simulink model "BALLBOT_2"  (R2015a)
settings: Solver=ode45  SolverMode=SingleTasking  StartTime=0  StopTime=90  MaxStep=0.001  RelTol=1e-3  AbsTol=1e-6
InitFcn:
  | parametros;
StartFcn:
  | %vrview('Ballbot2')
StopFcn:
  | graficos;
values from neighbouring files (symbols this model uses):
  g = 9.81    [parametros.m]
  Ic = 0.024    [parametros.m]
  L = 0.2    [parametros.m]
  Mc = 1.6    [parametros.m]
  Mr = 0.5    [parametros.m]
  r = 0.12    [parametros.m]
undefined symbols (not defined in the file or in its folder): K
libraries: vrlib x4, mblibv1 x1
settings Model: ExtModeAutoUpdateStatusClock=off  Creator=The MathWorks Inc.  LastModifiedBy=Pedro
settings DataIOCC: ExternalInput=[]  InitialState=[]  LimitDataPoints=off  SignalLoggingSaveFormat=ModelDataLogs  SaveOutput=off  SaveTime=off
settings OptimizationCC: BlockReduction=off  BooleanDataType=off  BufferReuse=off  ExpressionDepthLimit=2147483647  InitFltsAndDblsToZero=on
settings DebuggingCC: AlgebraicLoopMsg=none  SaveWithParameterizedLinksMsg=none  UnderspecifiedInitializationDetection=Classic  MergeDetectMultiDrivingBlocksExec=none  SignalResolutionControl=TryResolveAllWithWarning  MultiTaskDSMMsg=warning  MultiTaskCondExecSysMsg=none  SigSpecEnsureSampleTimeMsg=none  FcnCallInpInsideContextMsg=UseLocalSettings  UnconnectedInputMsg=none  UnconnectedOutputMsg=none  UnconnectedLineMsg=none  StateNameClashWarn=warning
settings HardwareCC: TargetLongLongMode=on  TargetIntDivRoundTo=Zero  TargetEndianess=LittleEndian  TargetHWDeviceType=MATLAB Host  ProdEqTarget=off
settings GRTTargetCC: TargetFcnLib=ansi_tfl_tmw.mat  CombineOutputUpdateFcns=off  GRTInterface=on

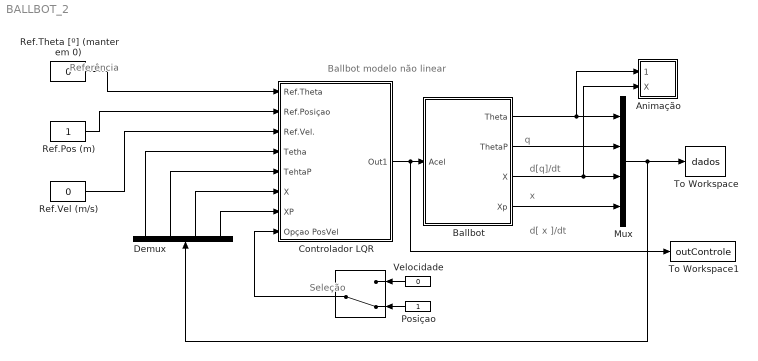
== system BALLBOT_2 ==
  note: Ballbot modelo não linear
  note: Referência
  note: Seleção
  note: x
  note: d[ x ]/dt
  note: q
  note: d[q]/dt
  " " : ManualSwitch  CurrentSetting=0
  "Animação " : Subsystem
  Ballbot : Subsystem  mask(Ballbot){thetac0=0}
      mask prompts: thetac0 "Ângulo inicial do corpo (graus)"
      mask help:
      | Modelo dinâmico não-linear do Ballbot.
      | Selecione "Look Under Mask" para ver o diagrama de simulação.
      mask Help: Unmask and double-click to see dynamics.
      mask Display: image(imread('ballbot_LMI.png'));
  Controlador LQR : Subsystem
      mask Display:
      | image(imread('ArduinoMega.png'));
      | 
      | 
      | 
      | port_label('output', 1, 'Acel Ang.');
      | 
      | port_label('input', 1, 'Ref.Theta');
      | port_label('input', 2, 'Ref.Pos.');
      | port_label('input', 3, 'Ref.Vel.');
      | port_label('input', 4, 'Theta');
      | port_label('input', 5, 'ThetaP');
      | port_label('input', 6, 'X');
      | port_label('input', 7, 'XP');
      | 
      | port_label('input', 8, 'Opção Pos.Vel');
  Demux : Demux
  Mux : Mux
  Posiçao : Constant
  "Ref.Pos (m) " : Constant
  Ref.Theta [º] (manter em 0) : Constant  Value=0
  Ref.Vel (m/s) : Constant  Value=0
  To Workspace : ToWorkspace  VariableName=dados  SaveFormat=Structure With Time  SampleTime=-1
  To Workspace1 : ToWorkspace  VariableName=outControle  SaveFormat=Structure With Time  SampleTime=-1
  Velocidade : Constant  Value=0
  wires:
  Ballbot/1(Theta) -> "Animação "/1("Pitch "), Mux/1
  Ballbot/2(ThetaP) -> Mux/2
  Ballbot/4(Xp) -> Mux/4
  Ref.Theta [º] (manter em 0)/1 -> Controlador LQR/1(Ref.Theta)
  Ref.Vel (m/s)/1 -> Controlador LQR/3(Ref.Vel.)
  Demux/1 -> Controlador LQR/4(Tetha)
  Demux/2 -> Controlador LQR/5(TehtaP)
  Demux/3 -> Controlador LQR/6(X)
  Demux/4 -> Controlador LQR/7(XP)
  Mux/1 -> Demux/1, To Workspace/1
  Velocidade/1 -> " "/1
  Posiçao/1 -> " "/2
  " "/1 -> Controlador LQR/8(Opçao PosVel)
  "Ref.Pos (m) "/1 -> Controlador LQR/2(Ref.Posiçao)
  Controlador LQR/1(Out1) -> To Workspace1/1, Ballbot/1(Acel)
  Ballbot/3(X) -> "Animação "/2(X), Mux/3

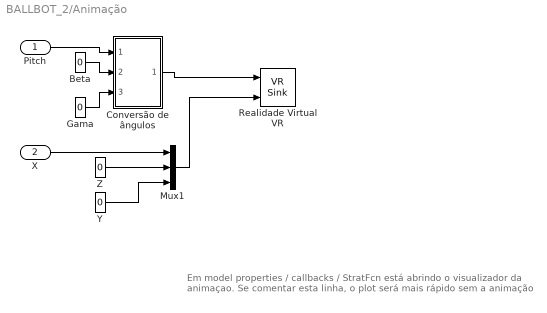
== system BALLBOT_2/Animação  ==
  note: Em model properties / callbacks / StratFcn está abrindo o visualizador da animaçao. Se comentar esta linha, o plot será mais rápido sem a animação
  "Pitch " : Inport
  X : Inport  Port=2
  Beta : Constant  Value=0
  Conversão de ângulos : Subsystem
  Gama : Constant  Value=0
  Mux1 : Mux  Inputs=3
  Realidade Virtual VR : vrlib/VR Sink  InstantiateOnLoad=on  SampleTime=0.001  ViewEnable=on  RemoteChange=off  RemoteView=off  FieldsWritten=Ballbot.rotation.4.1.1.double#Ballbot.translation.3.1.1.double  WorldFileName=Ballbot2.WRL  AutoView=on  VideoDimensions=[]  AllowVariableSize=off  FigureProperties="{'Position', 'Name', 'Viewpoint', 'CameraBound', 'CameraDirection', 'CameraPosition', 'CameraUpVector', 'ZoomFactor', 'Antialiasing', 'Headlight', 'Lighting', 'NavPanel', 'Sound', 'StatusBar', 'Stereo3D', 'Stereo3DCameraOffset', 'Stereo3DHIT', 'ToolBar', 'Textures', 'Transparency', 'Triad', 'Wireframe', 'NavZones', 'NavMode', 'NavSpeed', 'CaptureFileFormat', 'CaptureFileName', 'Record2DCompressMethod', 'Record2DCompressQuality', 'Record2D', 'Record2DFileName', 'Record2DFPS'; [5.0000000000000000e+00   9.2000000000000000e+01   5.7600000000000000e+02   3.8000000000000000e+02], '', '_untitled_1', 'on', [0.0000000000000000e+00   0.0000000000000000e+00  -1.0000000000000000e+00], [0.0000000000000000e+00   0.0000000000000000e+00   0.0000000000000000e+00], [0.0000000000000000e+00   1.0000000000000000e+00   0.0000000000000000e+00], [1.0000000000000000e+00], 'on', 'on', 'on', 'halfbar', 'on', 'on', 'off', [1.0000000149011612e-01], [0.0000000000000000e+00], 'on', 'on', 'on', 'none', 'off', 'off', 'fly', 'normal', 'tif', '%f_anim_%n.tif', 'auto', [7.5000000000000000e+01], 'off', '%f_anim_%n.avi', 'auto'}"
  Y : Constant  Value=0
  Z : Constant  Value=0
  wires:
  Z/1 -> Mux1/2
  Conversão de ângulos/1(Saida) -> Realidade Virtual VR/1
  Mux1/1 -> Realidade Virtual VR/2
  Beta/1 -> Conversão de ângulos/2(Beta)
  Gama/1 -> Conversão de ângulos/3(Gama)
  Y/1 -> Mux1/3
  X/1 -> Mux1/1
  "Pitch "/1 -> Conversão de ângulos/1(Alfa)

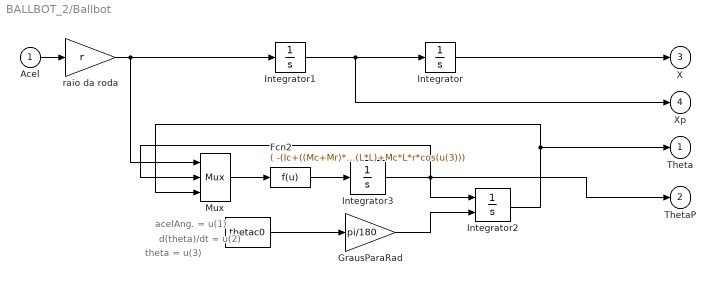
== system BALLBOT_2/Ballbot ==
  note: theta = u(3)
  note: d(theta)/dt = u(2)
  note: acelAng. = u(1)
  Acel : Inport
  "   " : Constant  Value=thetac0
  Fcn2 : Fcn  Expr=( -(Ic+((Mc+Mr)*r*r)+Mc*L*r*cos(u(3)))*u(1) + Mc*g*L*sin(u(3))+Mc*r*L*u(2)*u(2)*sin(u(3)))/ (Ic+Mc*(L*L)+Mc*L*r*cos(u(3)))
  "GrausParaRad " : Gain  Gain=pi/180
  Integrator : Integrator
  Integrator1 : Integrator
  Integrator2 : Integrator  InitialConditionSource=external
  Integrator3 : Integrator
  Mux : Mux  Inputs=3
  raio da roda : Gain  Gain=r
  Theta : Outport
  ThetaP : Outport  Port=2
  X : Outport  Port=3
  Xp : Outport  Port=4
  wires:
  Fcn2/1 -> Integrator3/1
  Mux/1 -> Fcn2/1
  Integrator2/1 -> Mux/3, Theta/1
  "   "/1 -> "GrausParaRad "/1
  "GrausParaRad "/1 -> Integrator2/2
  Integrator3/1 -> Mux/2, ThetaP/1, Integrator2/1
  Integrator/1 -> X/1
  Integrator1/1 -> Xp/1, Integrator/1
  Acel/1 -> raio da roda/1
  raio da roda/1 -> Integrator1/1, Mux/1

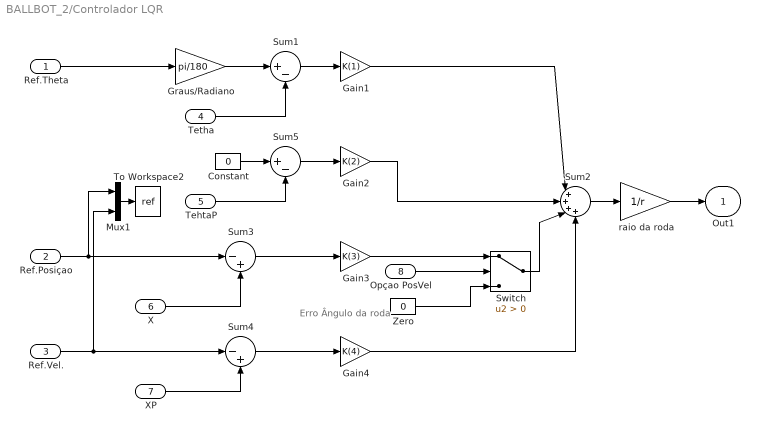
== system BALLBOT_2/Controlador LQR ==
  note: Erro
      | Ângulo da roda
  Ref.Theta : Inport
  Ref.Posiçao : Inport  Port=2
  Ref.Vel. : Inport  Port=3
  Tetha : Inport  Port=4
  TehtaP : Inport  Port=5
  X : Inport  Port=6
  XP : Inport  Port=7
  Opçao PosVel : Inport  Port=8
  Constant : Constant  Value=0
  Gain1 : Gain  Gain=K(1)
  Gain2 : Gain  Gain=K(2)
  Gain3 : Gain  Gain=K(3)
  Gain4 : Gain  Gain=K(4)
  Graus/Radiano : Gain  Gain=pi/180
  Mux1 : Mux  Inputs=2
  Sum1 : Sum  Inputs=|+-
  Sum2 : Sum  Inputs=|++++
  Sum3 : Sum  Inputs=|-+
  Sum4 : Sum  Inputs=|-+
  Sum5 : Sum  Inputs=|+-
  Switch : Switch  Criteria=u2 > Threshold
  To Workspace2 : ToWorkspace  VariableName=ref  SaveFormat=Structure With Time  SampleTime=-1
  Zero : Constant  Value=0
  raio da roda : Gain  Gain=1/r
  Out1 : Outport
  wires:
  Gain1/1 -> Sum2/1
  Gain2/1 -> Sum2/2
  Gain4/1 -> Sum2/4
  Ref.Theta/1 -> Graus/Radiano/1
  Tetha/1 -> Sum1/2
  Sum1/1 -> Gain1/1
  Graus/Radiano/1 -> Sum1/1
  Opçao PosVel/1 -> Switch/2
  Gain3/1 -> Switch/1
  Switch/1 -> Sum2/3
  Zero/1 -> Switch/3
  Sum5/1 -> Gain2/1
  TehtaP/1 -> Sum5/2
  Constant/1 -> Sum5/1
  X/1 -> Sum3/2
  XP/1 -> Sum4/2
  Sum3/1 -> Gain3/1
  Sum4/1 -> Gain4/1
  Ref.Vel./1 -> Mux1/2, Sum4/1
  Ref.Posiçao/1 -> Mux1/1, Sum3/1
  Mux1/1 -> To Workspace2/1
  Sum2/1 -> raio da roda/1
  raio da roda/1 -> Out1/1

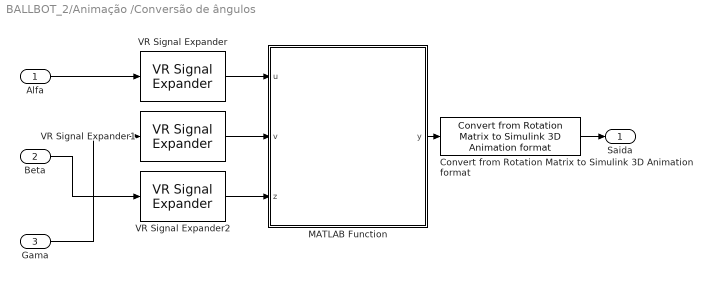
== system BALLBOT_2/Animação /Conversão de ângulos ==
  Alfa : Inport
  Beta : Inport  Port=2
  Gama : Inport  Port=3
  Convert from Rotation Matrix to Simulink 3D Animation format : mblibv1/Utilities/Convert from Rotation Matrix to Simulink 3D Animation format
  MATLAB Function : MATLAB Function  TreatAsAtomicUnit=on
  VR Signal Expander : vrlib/VR Signal Expander  outwidth=1  outidx=1
  VR Signal Expander1 : vrlib/VR Signal Expander  outwidth=1  outidx=1
  VR Signal Expander2 : vrlib/VR Signal Expander  outwidth=1  outidx=1
  Saida : Outport
  wires:
  Beta/1 -> VR Signal Expander2/1
  Gama/1 -> VR Signal Expander1/1
  VR Signal Expander1/1 -> MATLAB Function/2(v)
  Alfa/1 -> VR Signal Expander/1
  VR Signal Expander/1 -> MATLAB Function/1(u)
  MATLAB Function/1(y) -> Convert from Rotation Matrix to Simulink 3D Animation format/1
  Convert from Rotation Matrix to Simulink 3D Animation format/1 -> Saida/1
  VR Signal Expander2/1 -> MATLAB Function/3(z)

== matlab function BALLBOT_2/Animação /Conversão de ângulos/MATLAB Function ==
  data: u input; y output; v input; z input
function y = fcn(u,v,z)
%#codegen
temp=eul2rotm([u v z]);
saida=[temp(1,:) temp(2,:) temp(3,:)];
y = saida;
end
